simulink model "lab0"  (R2022b)
settings: Solver=VariableStepAuto  StartTime=0.0  StopTime=10.0  RelTol=1e-3
values from neighbouring files (symbols this model uses):
  der =     [parameters 2.mat]    (also in parameters.mat)
  drv =     [parameters 2.mat]    (also in parameters.mat)
  gbox =     [parameters 2.mat]    (also in parameters.mat)
  mld =     [parameters 2.mat]    (also in parameters.mat)
  mot =     [parameters 2.mat]    (also in parameters.mat)
  pid =     [parameters 2.mat]    (also in parameters.mat)
  rads2rpm = 60/2/pi    (= 9.54929658551)    [load_params_inertial_case.m]    (also in parameters 2.mat; parameters.mat)
  sens =     [parameters 2.mat]    (also in parameters.mat)
  Ts = 1e-3    (= 0.001)    [load_params_inertial_case.m]    (also in parameters 2.mat; parameters.mat)
settings Model: Creator=emanuelevitetta  LastModifiedBy=emanuelevitetta

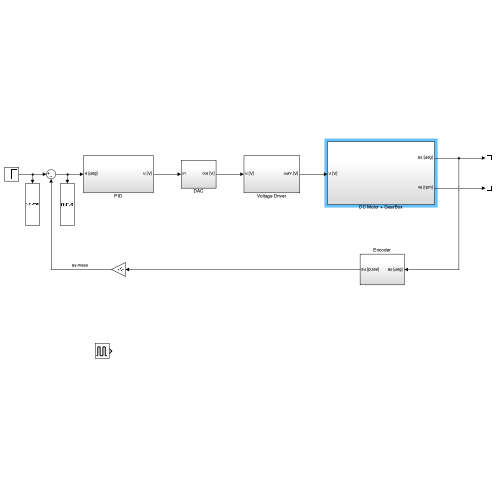
[thumbnail: Simulink's stored preview of the top-level diagram]
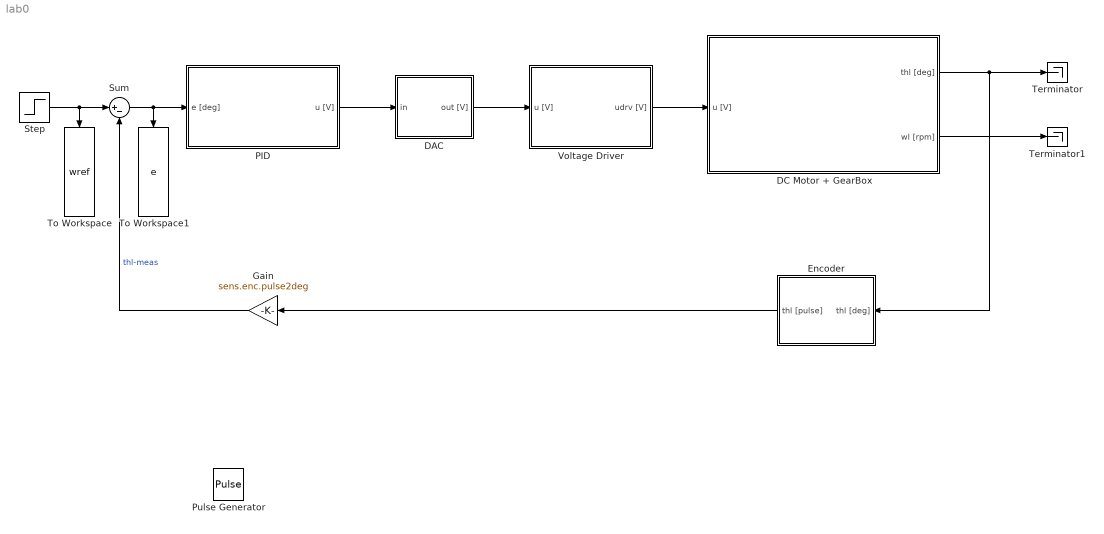
== system lab0 ==
  DAC : Subsystem
  DC Motor + GearBox : Subsystem
  Encoder : Subsystem
  Gain : Gain  Gain=sens.enc.pulse2deg
  PID : Subsystem
  Pulse Generator : DiscretePulseGenerator  PulseType=Time based  Period=10  PulseWidth=5
  Step : Step  After=10  SampleTime=0
  Sum : Sum  Inputs=|+-
  Terminator : Terminator
  Terminator1 : Terminator
  To Workspace : ToWorkspace  VariableName=wref  SaveFormat=Timeseries  SampleTime=-1
  To Workspace1 : ToWorkspace  VariableName=e  SaveFormat=Timeseries  SampleTime=-1
  Voltage Driver : Subsystem
  wires:
  DC Motor + GearBox/1(thl [deg]) -> Encoder/1(thl [deg]), Terminator/1
  DC Motor + GearBox/2(wl [rpm]) -> Terminator1/1
  Voltage Driver/1(udrv [V]) -> DC Motor + GearBox/1(u [V])
  DAC/1(out [V]) -> Voltage Driver/1(u [V])
  PID/1(u [V]) -> DAC/1(in)
  Encoder/1(thl [pulse]) -> Gain/1
  Sum/1 -> To Workspace1/1, PID/1(e [deg])
  Gain/1 -> Sum/2  "thl-meas"
  Step/1 -> To Workspace/1, Sum/1

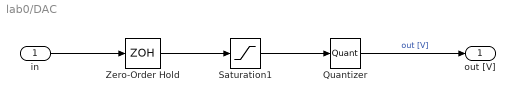
== system lab0/DAC ==
  in : Inport
  Quantizer : Quantizer  QuantizationInterval=daq.dac.q
  Saturation1 : Saturate  UpperLimit=10  LowerLimit=-10
  Zero-Order Hold : ZeroOrderHold  SampleTime=Ts
  out [V] : Outport
  wires:
  Quantizer/1 -> out [V]/1  "out [V]"
  in/1 -> Zero-Order Hold/1
  Zero-Order Hold/1 -> Saturation1/1
  Saturation1/1 -> Quantizer/1

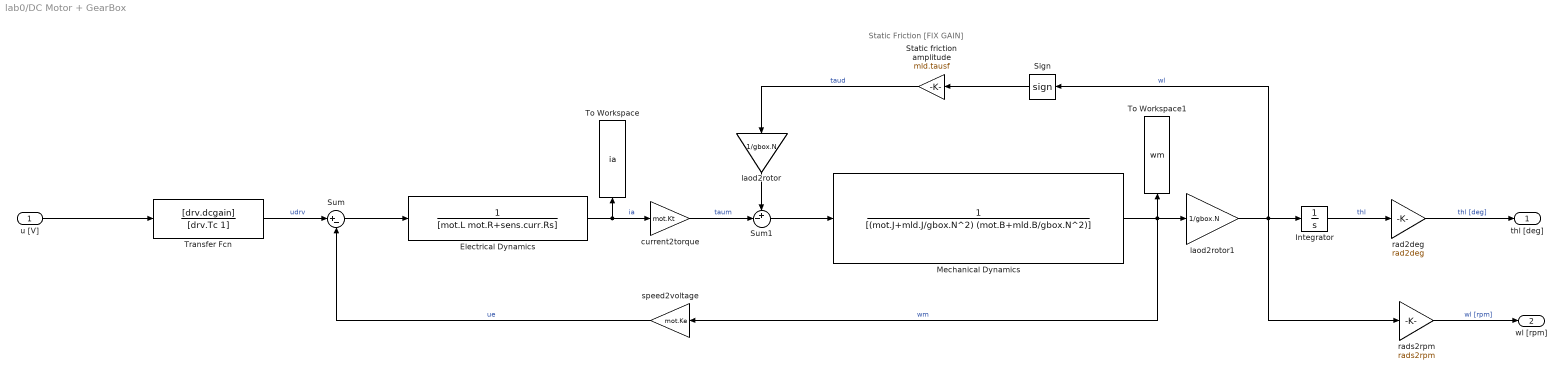
== system lab0/DC Motor + GearBox ==
  note: Static Friction [FIX GAIN]
  u [V] : Inport
  Electrical Dynamics : TransferFcn  Denominator=[mot.L mot.R+sens.curr.Rs]
  Integrator : Integrator
  Mechanical Dynamics : TransferFcn  Denominator=[(mot.J+mld.J/gbox.N^2) (mot.B+mld.B/gbox.N^2)]
  Sign : Signum  ZeroCross=off
  Static friction amplitude : Gain  Gain=mld.tausf
  Sum : Sum  Inputs=|+-
  Sum1 : Sum  Inputs=+-|
  To Workspace : ToWorkspace  VariableName=ia  SaveFormat=Timeseries  SampleTime=-1
  To Workspace1 : ToWorkspace  VariableName=wm  SaveFormat=Timeseries  SampleTime=-1
  Transfer Fcn : TransferFcn  Numerator=[drv.dcgain]  Denominator=[drv.Tc 1]
  current2torque : Gain  Gain=mot.Kt
  laod2rotor : Gain  Gain=1/gbox.N
  laod2rotor1 : Gain  Gain=1/gbox.N
  rad2deg : Gain  Gain=rad2deg
  rads2rpm : Gain  Gain=rads2rpm
  speed2voltage : Gain  Gain=mot.Ke
  thl [deg] : Outport
  wl [rpm] : Outport  Port=2
  wires:
  rads2rpm/1 -> wl [rpm]/1  "wl [rpm]"
  u [V]/1 -> Transfer Fcn/1
  Sign/1 -> Static friction amplitude/1
  Electrical Dynamics/1 -> To Workspace/1, current2torque/1  "ia"
  Sum1/1 -> Mechanical Dynamics/1
  laod2rotor1/1 -> rads2rpm/1, Sign/1, Integrator/1  "wl"
  rad2deg/1 -> thl [deg]/1  "thl [deg]"
  laod2rotor/1 -> Sum1/1
  Transfer Fcn/1 -> Sum/1  "udrv"
  current2torque/1 -> Sum1/2  "taum"
  Static friction amplitude/1 -> laod2rotor/1  "taud"
  speed2voltage/1 -> Sum/2  "ue"
  Integrator/1 -> rad2deg/1  "thl"
  Sum/1 -> Electrical Dynamics/1
  Mechanical Dynamics/1 -> laod2rotor1/1, To Workspace1/1, speed2voltage/1  "wm"

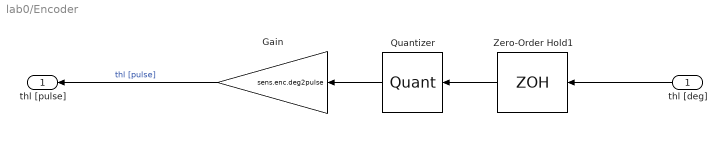
== system lab0/Encoder ==
  thl [deg] : Inport
  Gain : Gain  Gain=sens.enc.deg2pulse
  Quantizer : Quantizer
  Zero-Order Hold1 : ZeroOrderHold  SampleTime=Ts
  thl [pulse] : Outport
  wires:
  thl [deg]/1 -> Zero-Order Hold1/1
  Zero-Order Hold1/1 -> Quantizer/1
  Gain/1 -> thl [pulse]/1  "thl [pulse]"
  Quantizer/1 -> Gain/1

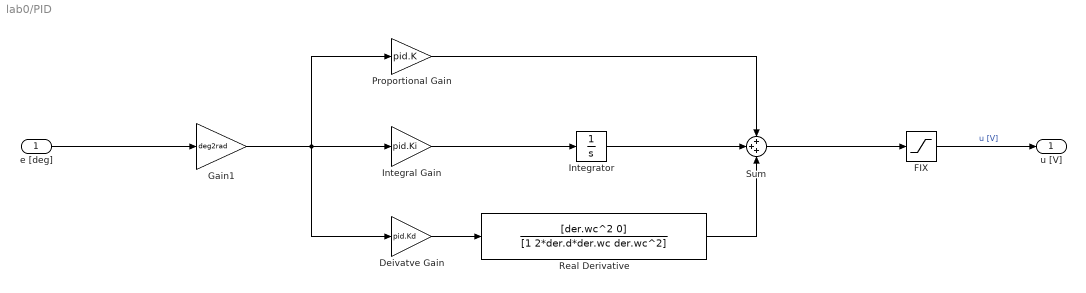
== system lab0/PID ==
  e [deg] : Inport
  Deivatve Gain : Gain  Gain=pid.Kd
  "FIX " : Saturate
  Gain1 : Gain  Gain=deg2rad
  Integral Gain : Gain  Gain=pid.Ki
  Integrator : Integrator
  Proportional Gain : Gain  Gain=pid.K
  Real Derivative : TransferFcn  Numerator=[der.wc^2 0]  Denominator=[1 2*der.d*der.wc der.wc^2]
  Sum : Sum  Inputs=+++
  u [V] : Outport
  wires:
  Deivatve Gain/1 -> Real Derivative/1
  e [deg]/1 -> Gain1/1
  Integrator/1 -> Sum/2
  "FIX "/1 -> u [V]/1  "u [V]"
  Gain1/1 -> Deivatve Gain/1, Proportional Gain/1, Integral Gain/1
  Real Derivative/1 -> Sum/3
  Integral Gain/1 -> Integrator/1
  Proportional Gain/1 -> Sum/1
  Sum/1 -> "FIX "/1

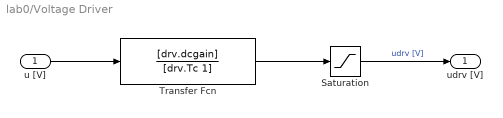
== system lab0/Voltage Driver ==
  u [V] : Inport
  Saturation : Saturate  UpperLimit=12  LowerLimit=-12
  Transfer Fcn : TransferFcn  Numerator=[drv.dcgain]  Denominator=[drv.Tc 1]
  udrv [V] : Outport
  wires:
  Saturation/1 -> udrv [V]/1  "udrv [V]"
  u [V]/1 -> Transfer Fcn/1
  Transfer Fcn/1 -> Saturation/1
